simulink model "geometric_control_template"  (R2025b)
settings: Solver=VariableStepAuto  StartTime=0.0  StopTime=30.0  RelTol=1e-3
InitFcn:
  | %% INITIALIZATION
  | 
  | clearvars -except out
  | clc
  | 
  | %% UAV PARAMETERS
  | 
  | mass = 1.2;        % [kg] mass used by controllers
  | mass_real = 1.2;  % [kg] mass used by dynamics
  | 
  | Ib = diag([1.2416 1.2416 2*1.2416]);
  | Ib_ctrl = diag([1.0 0.85 1.80]);
  | %Ib_ctrl = diag([1.2416 1.2416 2*1.2416]);
  | %% SAMPLING TIME
  | 
  | Ts = 0.001;
  | 
  | %% PLANNER
  | 
  | t_iniz = 0;
  | ttot = 22;       % trajectory duration [s]
  | tdead = 8;       % final steady-state time [s]
  | tot_time = ttot + tdead;
  | 
  | % Include exactly t = ttot
  | t1 = 0:Ts:ttot;
  | t_dead = (ttot+Ts):Ts:tot_time;
  | t = [t1, t_dead];
  | 
  | N1 = length(t1);
  | Ndead = length(t_dead);
  | 
  | %% INITIAL CONDITIONS
  | 
  | x0 = 0;
  | y0 = 0;
  | z0 = -1;
  | psi0 = 0;
  | 
  | x0_real = x0;
  | y0_real = y0;
  | z0_real = z0;
  | 
  | pos_0 = [x0_real y0_real z0_real];
  | lin_vel_0 = [0 0 0];
  | w_bb_0 = [0 0 0];
  | 
  | %% SMOOTH NORMALIZED TIME
  | 
  | sigma = t1 / ttot;
  | 
  | % 7th-order smooth step:
  | % s(0)=0, s(1)=1
  | % sdot(0)=sdot(1)=0
  | % sddot(0)=sddot(1)=0
  | % sdddot(0)=sdddot(1)=0
  | 
  | s = 35*sigma.^4 - 84*sigma.^5 + 70*sigma.^6 - 20*sigma.^7;
  | 
  | sdot = (140*sigma.^3 ...
  |       - 420*sigma.^4 ...
  |       + 420*sigma.^5 ...
  |       - 140*sigma.^6) / ttot;
  | 
  | sddot = (420*sigma.^2 ...
  |        - 1680*sigma.^3 ...
  |        + 2100*sigma.^4 ...
  |        - 840*sigma.^5) / ttot^2;
  | 
  | %% DESIRED TRAJECTORY PARAMETERS
  | 
  | Dx = 1.20;
  | Dy = 0.70;
  | Dz = -1.70;
  | 
  | Ay_bump = 0.35;
  | Az_bump = 0.18;
  | 
  | psi_final = deg2rad(25);
  | psi_bump  = deg2rad(6);
  | 
  | %% DESIRED POSITION
  | 
  | x_d = x0 + Dx*s;
  | 
  | y_d = y0 + Dy*s + Ay_bump*sin(2*pi*s);
  | 
  | z_d = z0 + Dz*s + Az_bump*sin(pi*s);
  | 
  | psi_d_traj = psi0 + psi_final*s + psi_bump*sin(pi*s);
  | 
  | %% DERIVATIVES WITH RESPECT TO s
  | 
  | x_s = Dx;
  | x_ss = 0;
  | 
  | y_s = Dy + Ay_bump*2*pi*cos(2*pi*s);
  | y_ss = -Ay_bump*(2*pi)^2*sin(2*pi*s);
  | 
  | z_s = Dz + Az_bump*pi*cos(pi*s);
  | z_ss = -Az_bump*pi^2*sin(pi*s);
  | 
  | psi_s = psi_final + psi_bump*pi*cos(pi*s);
  | psi_ss = -psi_bump*pi^2*sin(pi*s);
  | 
  | %% DESIRED VELOCITY
  | 
  | dot_x_d = x_s .* sdot;
  | dot_y_d = y_s .* sdot;
  | dot_z_d = z_s .* sdot;
  | 
  | dot_psi_d_traj = psi_s .* sdot;
  | 
  | %% DESIRED ACCELERATION
  | 
  | ddot_x_d = x_ss .* sdot.^2 + x_s .* sddot;
  | ddot_y_d = y_ss .* sdot.^2 + y_s .* sddot;
  | ddot_z_d = z_ss .* sdot.^2 + z_s .* sddot;
  | 
  | ddot_psi_d_traj = psi_ss .* sdot.^2 + psi_s .* sddot;
  | 
  | %% ADD FINAL STEADY-STATE PART
  | 
  | x_final = x_d(end);
  | y_final = y_d(end);
  | z_final = z_d(end);
  | psi_final_value = psi_d_traj(end);
  | 
  | p_d = zeros(4, length(t));
  | dot_p_d = zeros(4, length(t));
  | ddot_p_d = zeros(4, length(t));
  | 
  | p_d(1,:) = [x_d, x_final*ones(1, Ndead)];
  | p_d(2,:) = [y_d, y_final*ones(1, Ndead)];
  | p_d(3,:) = [z_d, z_final*ones(1, Ndead)];
  | p_d(4,:) = [psi_d_traj, psi_final_value*ones(1, Ndead)];
  | 
  | dot_p_d(1,:) = [dot_x_d, zeros(1, Ndead)];
  | dot_p_d(2,:) = [dot_y_d, zeros(1, Ndead)];
  | dot_p_d(3,:) = [dot_z_d, zeros(1, Ndead)];
  | dot_p_d(4,:) = [dot_psi_d_traj, zeros(1, Ndead)];
  | 
  | ddot_p_d(1,:) = [ddot_x_d, zeros(1, Ndead)];
  | ddot_p_d(2,:) = [ddot_y_d, zeros(1, Ndead)];
  | ddot_p_d(3,:) = [ddot_z_d, zeros(1, Ndead)];
  | ddot_p_d(4,:) = [ddot_psi_d_traj, zeros(1, Ndead)];
  | 
  | %% DATA FOR SIMULINK
  | 
  | csi_d = p_d(1:3,:);
  | dot_csi_d = dot_p_d(1:3,:);
  | ddot_csi_d = ddot_p_d(1:3,:);
  | 
  | psi_d = p_d(4,:);
  | dot_psi_d = dot_p_d(4,:);
  | ddot_psi_d = ddot_p_d(4,:);
  | 
  | %% DESIRED BODY X-AXIS FROM YAW
  | 
  | xb_des = zeros(3, length(t));
  | 
  | xb_des(1,:) = cos(psi_d);
  | xb_des(2,:) = sin(psi_d);
  | xb_des(3,:) = zeros(1, length(t));
  | 
  | %% EXTERNAL FORCE DISTURBANCE
  | 
  | f_ext = zeros(length(t), 3);
  | 
  | t_f_on = 8;
  | t_f_off = 14;
  | 
  | f_ex_amp = 1.0;    % [N]
  | f_ey_amp = 1.0;    % [N]
  | f_ez_amp = 1.0;    % [N]
  | 
  | t_smooth_f = 0.3;  % [s] smoothing time
  | 
  | w_on_f  = 0.5 * (1 + tanh((t - t_f_on)/t_smooth_f));
  | w_off_f = 0.5 * (1 - tanh((t - t_f_off)/t_smooth_f));
  | 
  | dist_window_f = w_on_f .* w_off_f;
  | 
  | f_ext(:,1) = f_ex_amp * dist_window_f(:);
  | f_ext(:,2) = f_ey_amp * dist_window_f(:);
  | f_ext(:,3) = f_ez_amp * dist_window_f(:);
  | 
  | f_ext_ts = timeseries(f_ext, t(:));
  | 
  | %% EXTERNAL TORQUE DISTURBANCE
  | 
  | tau_ext = zeros(length(t), 3);
  | 
  | t_tau_on = 8;
  | t_tau_off = 14;
  | 
  | tau_ex_amp = 0.0;    % [Nm]
  | tau_ey_amp = 0.5;    % [Nm]
  | tau_ez_amp = 0.0;    % [Nm]
  | 
  | t_smooth_tau = 0.3;  % [s] smoothing time
  | 
  | w_on_tau  = 0.5 * (1 + tanh((t - t_tau_on)/t_smooth_tau));
  | w_off_tau = 0.5 * (1 - tanh((t - t_tau_off)/t_smooth_tau));
  | 
  | dist_window_tau = w_on_tau .* w_off_tau;
  | 
  | tau_ext(:,1) = tau_ex_amp * dist_window_tau(:);
  | tau_ext(:,2) = tau_ey_amp * dist_window_tau(:);
  | tau_ext(:,3) = tau_ez_amp * dist_window_tau(:);
  | 
  | tau_ext_ts = timeseries(tau_ext, t(:));
  | 
  | 
  | %% CHECK
  | 
  | disp("InitFcn completed.")
  | disp("mass = " + string(mass) + " kg")
  | disp("mass_real = " + string(mass_real) + " kg")
  | disp("Simulation time = " + string(tot_time) + " s")
  | disp("Force disturbance: [" + string(f_ex_amp) + ", " + string(f_ey_amp) + ", " + string(f_ez_amp) + "] N")
  | disp("Torque disturbance: [" + string(tau_ex_amp) + ", " + string(tau_ey_amp) + ", " + string(tau_ez_amp) + "] Nm")
undefined symbols (not defined in the file or in its folder): dspblkCoreblockFVToolHelper, gcbh
libraries: robotcorelib x1
settings Model: Creator=fabioruggiero  LastModifiedBy=miche
settings ModelReferenceCC: EnableRefExpFcnMdlSchedulingChecks=on
settings RTWCC: GPUComputeCapability=3.5

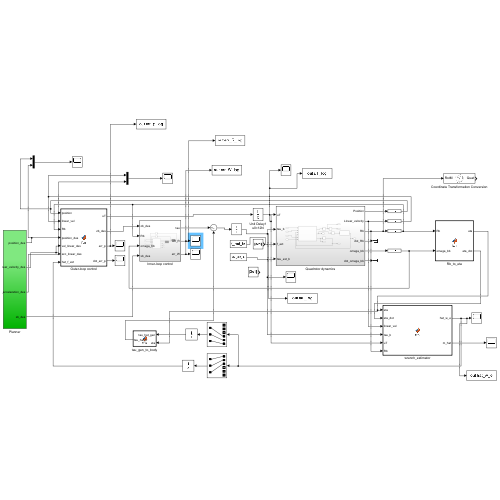
[thumbnail: Simulink's stored preview of the top-level diagram]
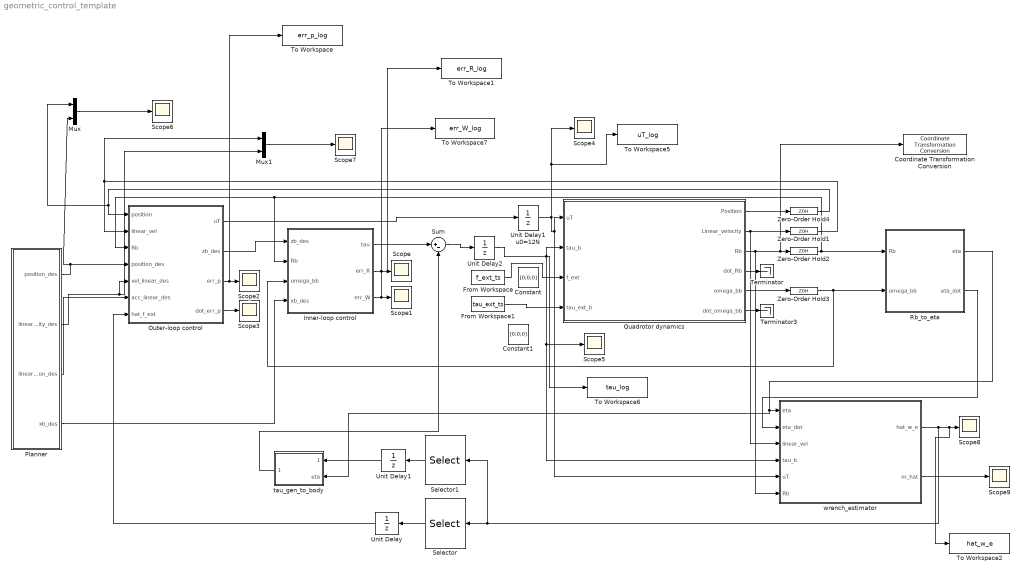
== system geometric_control_template ==
  Constant : Constant  Value=[0;0;0]
  Constant1 : Constant  Value=[0;0;0]
  Coordinate Transformation Conversion : robotcorelib/Coordinate Transformation Conversion  InputRepresentation=Rotation Matrix  InputEulerSequence=ZYX  ShowTrVecInputPort=on  OutputRepresentation=Quaternion  OutputEulerSequence=ZYX  ShowTrVecOutputPort=on  SimulateUsing=Interpreted execution
  From Workspace : FromWorkspace  VariableName=f_ext_ts
  From Workspace1 : FromWorkspace  VariableName=tau_ext_ts
  Inner-loop control : Subsystem
  Mux : Mux  Inputs=2
  Mux1 : Mux  Inputs=2
  Outer-loop control : MATLAB Function  TreatAsAtomicUnit=on
  Planner : Subsystem
  Quadrotor dynamics : Subsystem
  Rb_to_eta : MATLAB Function  TreatAsAtomicUnit=on
  Scope{,1..9} (10 alike) : Scope
      Scope settings: ActiveDisplayYMinimum=-0.020550467345848471  ActiveDisplayYMaximum=0.019993718220872751
      Scope1 settings: ActiveDisplayYMinimum=-0.00025864687025991271  ActiveDisplayYMaximum=0.00043427054129709314
      Scope2 settings: ActiveDisplayYMinimum=-0.0029648084696455505  ActiveDisplayYMaximum=0.02613326914388988  DataLoggingVariableName=ScopeData2
      Scope3 settings: ActiveDisplayYMinimum=-0.00022  ActiveDisplayYMaximum=8E-5  DataLoggingVariableName=ScopeData3
      Scope4 settings: ActiveDisplayYMinimum=11.66747  ActiveDisplayYMaximum=12.03695  DataLoggingVariableName=ScopeData4
      Scope5 settings: ActiveDisplayYMinimum=-5.4477992481437552  ActiveDisplayYMaximum=1.0297199075515178  DataLoggingVariableName=ScopeData5
      Scope6 settings: ActiveDisplayYMinimum=-8.59037  ActiveDisplayYMaximum=7.8245
      Scope7 settings: ActiveDisplayYMinimum=-0.38281946760904528  ActiveDisplayYMaximum=0.16406504710605604  DataLoggingVariableName=ScopeData2
      Scope8 settings: ActiveDisplayYMinimum=-0.0066285466449370889  ActiveDisplayYMaximum=0.0085233543920895938  DataLoggingVariableName=ScopeData6
      Scope9 settings: ActiveDisplayYMinimum=1.1924506191186222  ActiveDisplayYMaximum=1.2266627646008192  DataLoggingVariableName=ScopeData7
  Selector : Selector  InputPortWidth=6  IndexOptions=Index vector (dialog)  Indices=[1 2 3]  OutputSizes=1
  Selector1 : Selector  InputPortWidth=6  IndexOptions=Index vector (dialog)  Indices=[4 5 6]  OutputSizes=1
  Sum : Sum  Inputs=|+-
  Terminator : Terminator
  Terminator3 : Terminator
  To Workspace : ToWorkspace  VariableName=err_p_log  SaveFormat=Timeseries  SampleTime=Ts
  To Workspace1 : ToWorkspace  VariableName=err_R_log  SaveFormat=Timeseries  SampleTime=Ts
  To Workspace2 : ToWorkspace  VariableName=hat_w_e  SaveFormat=Timeseries  SampleTime=Ts
  To Workspace5 : ToWorkspace  VariableName=uT_log  SaveFormat=Timeseries  SampleTime=Ts
  To Workspace6 : ToWorkspace  VariableName=tau_log  SaveFormat=Timeseries  SampleTime=Ts
  To Workspace7 : ToWorkspace  VariableName=err_W_log  SaveFormat=Timeseries  SampleTime=Ts
  Unit Delay : UnitDelay  InitialCondition=[0; 0; 0]  SampleTime=-1  HasFrameUpgradeWarning=on
  Unit Delay1 : UnitDelay  InitialCondition=[0; 0; 0]  SampleTime=-1  HasFrameUpgradeWarning=on
  Unit Delay1 u0=12N : UnitDelay  InitialCondition=12  SampleTime=Ts
  Unit Delay2 : UnitDelay  InitialCondition=[0 0 0]  SampleTime=Ts
  Zero-Order Hold{1..4} (4 alike) : ZeroOrderHold  SampleTime=Ts
  tau_gen_to_body : MATLAB Function  TreatAsAtomicUnit=on
  wrench_estimator : MATLAB Function  TreatAsAtomicUnit=on
  wires:
  Outer-loop control/1(uT) -> Unit Delay1 u0=12N/1
  Unit Delay1 u0=12N/1 -> wrench_estimator/5(uT), Quadrotor dynamics/1(uT), To Workspace5/1, Scope4/1
  Quadrotor dynamics/1(Position) -> Zero-Order Hold4/1
  Quadrotor dynamics/2(Linear_velocity) -> wrench_estimator/3(linear_vel), Zero-Order Hold1/1
  Quadrotor dynamics/3(Rb) -> Coordinate Transformation Conversion/1, Zero-Order Hold2/1, wrench_estimator/6(Rb)
  Quadrotor dynamics/5(omega_bb) -> Zero-Order Hold3/1
  Zero-Order Hold2/1 -> Rb_to_eta/1(Rb), Outer-loop control/3(Rb), Inner-loop control/2(Rb)
  Quadrotor dynamics/4(dot_Rb) -> Terminator/1
  Planner/4(xb_des) -> Inner-loop control/4(xb_des)
  Outer-loop control/3(err_p) -> To Workspace/1, Scope2/1
  Outer-loop control/4(dot_err_p) -> Scope3/1
  Quadrotor dynamics/6(dot_omega_bb) -> Terminator3/1
  Outer-loop control/2(zb_des) -> Inner-loop control/1(zb_des)
  Zero-Order Hold3/1 -> Inner-loop control/3(omega_bb), Rb_to_eta/2(omega_bb)
  Inner-loop control/2(err_R) -> To Workspace1/1, Scope/1
  Inner-loop control/3(err_W) -> To Workspace7/1, Scope1/1
  Planner/1(position_des) -> Mux/2, Outer-loop control/4(position_des)
  Planner/2(linear_velocity_des) -> Mux1/2, Outer-loop control/5(vel_linear_des)
  Planner/3(linear_acceleration_des) -> Outer-loop control/6(acc_linear_des)
  Zero-Order Hold1/1 -> Outer-loop control/2(linear_vel), Mux1/1
  Zero-Order Hold4/1 -> Mux/1, Outer-loop control/1(position)
  Mux/1 -> Scope6/1
  Mux1/1 -> Scope7/1
  Rb_to_eta/1(eta) -> tau_gen_to_body/2(eta), wrench_estimator/1(eta)
  Rb_to_eta/2(eta_dot) -> wrench_estimator/2(eta_dot)
  Unit Delay2/1 -> To Workspace6/1, Quadrotor dynamics/2(tau_b), wrench_estimator/4(tau_b), Scope5/1
  wrench_estimator/2(m_hat) -> Scope9/1
  Selector1/1 -> Unit Delay1/1
  Selector/1 -> Unit Delay/1
  wrench_estimator/1(hat_w_e) -> To Workspace2/1, Scope8/1, Selector1/1, Selector/1
  Unit Delay1/1 -> tau_gen_to_body/1(tau_hat_gen)
  Inner-loop control/1(tau) -> Sum/1
  Sum/1 -> Unit Delay2/1
  From Workspace1/1 -> Quadrotor dynamics/4(tau_ext_b)
  From Workspace/1 -> Quadrotor dynamics/3(f_ext)
  Unit Delay/1 -> Outer-loop control/7(hat_f_ext)
  tau_gen_to_body/1(tau_hat_b) -> Sum/2

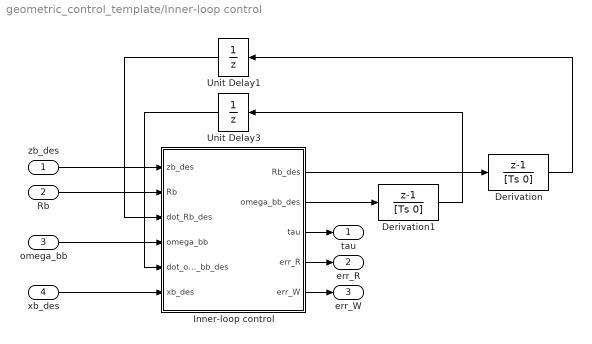
== system geometric_control_template/Inner-loop control ==
  zb_des : Inport
  Rb : Inport  Port=2
  omega_bb : Inport  Port=3
  xb_des : Inport  Port=4
  Derivation : DiscreteTransferFcn  LoadFcn=dspblkCoreblockFVToolHelper(gcbh,'load');  Numerator=[1 -1]  Denominator=[Ts 0]  InitialStates=[1 0 0;0 1 0;0 0 1]  SampleTime=Ts
      settings: CopyFcn=dspblkCoreblockFVToolHelper(gcbh,'copy');  DeleteFcn=dspblkCoreblockFVToolHelper(gcbh,'close');  ModelCloseFcn=dspblkCoreblockFVToolHelper(gcbh,'close');  PreSaveFcn=dspblkCoreblockFVToolHelper(gcbh,'presave');  PostSaveFcn=dspblkCoreblockFVToolHelper(gcbh,'postsave');  CloseFcn=dspblkCoreblockFVToolHelper(gcbh,'close');
  Derivation1 : DiscreteTransferFcn  Numerator=[1 -1]  Denominator=[Ts 0]  InitialStates=[0 0 0]  SampleTime=Ts
  Inner-loop control : MATLAB Function  TreatAsAtomicUnit=on
  Unit Delay1 : UnitDelay  InitialCondition=eye(3)  SampleTime=Ts
  Unit Delay3 : UnitDelay  InitialCondition=[0 0 0]  SampleTime=Ts
  tau : Outport
  err_R : Outport  Port=2
  err_W : Outport  Port=3
  wires:
  xb_des/1 -> Inner-loop control/6(xb_des)
  Inner-loop control/4(err_R) -> err_R/1
  Rb/1 -> Inner-loop control/2(Rb)
  Inner-loop control/3(tau) -> tau/1
  Unit Delay1/1 -> Inner-loop control/3(dot_Rb_des)
  Derivation1/1 -> Unit Delay3/1
  Inner-loop control/5(err_W) -> err_W/1
  Unit Delay3/1 -> Inner-loop control/5(dot_omega_bb_des)
  Derivation/1 -> Unit Delay1/1
  zb_des/1 -> Inner-loop control/1(zb_des)
  omega_bb/1 -> Inner-loop control/4(omega_bb)
  Inner-loop control/1(Rb_des) -> Derivation/1
  Inner-loop control/2(omega_bb_des) -> Derivation1/1

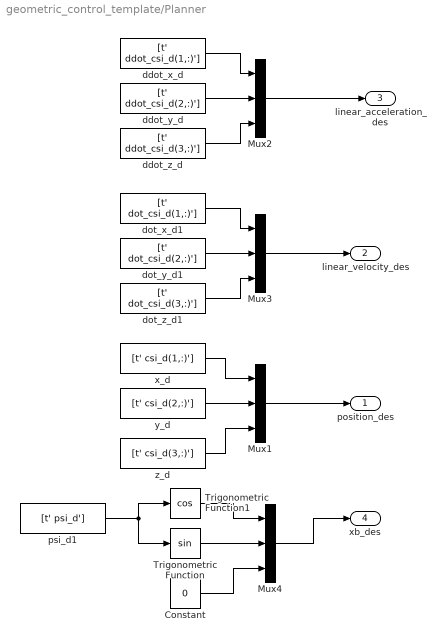
== system geometric_control_template/Planner ==
  Constant : Constant  Value=0
  Mux{1..4} (4 alike) : Mux  Inputs=3
  Trigonometric Function : Trigonometry
  Trigonometric Function1 : Trigonometry  Operator=cos
  ddot_x_d : FromWorkspace  VariableName=[t' ddot_csi_d(1,:)']  SampleTime=Ts
  ddot_y_d : FromWorkspace  VariableName=[t' ddot_csi_d(2,:)']  SampleTime=Ts
  ddot_z_d : FromWorkspace  VariableName=[t' ddot_csi_d(3,:)']  SampleTime=Ts
  dot_x_d1 : FromWorkspace  VariableName=[t' dot_csi_d(1,:)']  SampleTime=Ts
  dot_y_d1 : FromWorkspace  VariableName=[t' dot_csi_d(2,:)']  SampleTime=Ts
  dot_z_d1 : FromWorkspace  VariableName=[t' dot_csi_d(3,:)']  SampleTime=Ts
  psi_d1 : FromWorkspace  VariableName=[t' psi_d']  SampleTime=Ts
  x_d : FromWorkspace  VariableName=[t' csi_d(1,:)']  SampleTime=Ts
  y_d : FromWorkspace  VariableName=[t' csi_d(2,:)']  SampleTime=Ts
  z_d : FromWorkspace  VariableName=[t' csi_d(3,:)']  SampleTime=Ts
  position_des : Outport
  linear_velocity_des : Outport  Port=2
  linear_acceleration_des : Outport  Port=3
  xb_des : Outport  Port=4
  wires:
  y_d/1 -> Mux1/2
  z_d/1 -> Mux1/3
  x_d/1 -> Mux1/1
  ddot_y_d/1 -> Mux2/2
  ddot_z_d/1 -> Mux2/3
  ddot_x_d/1 -> Mux2/1
  Mux2/1 -> linear_acceleration_des/1
  Mux1/1 -> position_des/1
  dot_y_d1/1 -> Mux3/2
  dot_z_d1/1 -> Mux3/3
  dot_x_d1/1 -> Mux3/1
  Mux3/1 -> linear_velocity_des/1
  Mux4/1 -> xb_des/1
  Trigonometric Function/1 -> Mux4/2
  psi_d1/1 -> Trigonometric Function/1, Trigonometric Function1/1
  Trigonometric Function1/1 -> Mux4/1
  Constant/1 -> Mux4/3

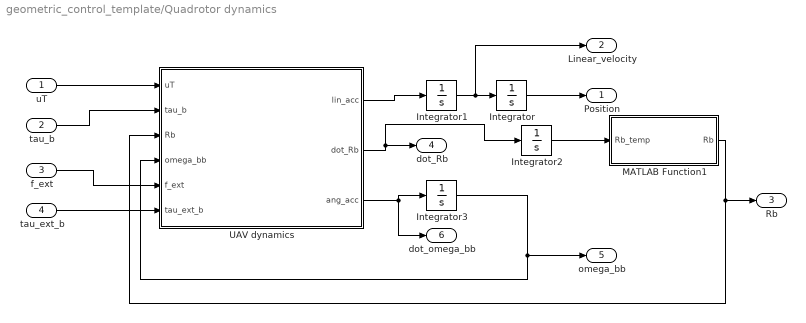
== system geometric_control_template/Quadrotor dynamics ==
  uT : Inport
  tau_b : Inport  Port=2
  f_ext : Inport  Port=3
  tau_ext_b : Inport  Port=4
  Integrator : Integrator  InitialCondition=pos_0
  Integrator1 : Integrator  InitialCondition=lin_vel_0
  Integrator2 : Integrator  InitialCondition=[1 0 0; 0 1 0;0 0 1]
  Integrator3 : Integrator  InitialCondition=w_bb_0
  MATLAB Function1 : MATLAB Function  TreatAsAtomicUnit=on
  UAV dynamics : MATLAB Function  TreatAsAtomicUnit=on
  Position : Outport
  Linear_velocity : Outport  Port=2
  Rb : Outport  Port=3
  dot_Rb : Outport  Port=4
  omega_bb : Outport  Port=5
  dot_omega_bb : Outport  Port=6
  wires:
  tau_b/1 -> UAV dynamics/2(tau_b)
  Integrator/1 -> Position/1
  UAV dynamics/3(ang_acc) -> Integrator3/1, dot_omega_bb/1
  UAV dynamics/1(lin_acc) -> Integrator1/1
  uT/1 -> UAV dynamics/1(uT)
  Integrator1/1 -> Linear_velocity/1, Integrator/1
  Integrator3/1 -> UAV dynamics/4(omega_bb), omega_bb/1
  UAV dynamics/2(dot_Rb) -> Integrator2/1, dot_Rb/1
  MATLAB Function1/1(Rb) -> Rb/1, UAV dynamics/3(Rb)
  Integrator2/1 -> MATLAB Function1/1(Rb_temp)
  f_ext/1 -> UAV dynamics/5(f_ext)
  tau_ext_b/1 -> UAV dynamics/6(tau_ext_b)

== matlab function geometric_control_template/Rb_to_eta ==
  data: Rb input; eta output; omega_bb input; eta_dot output
function [eta, eta_dot] = fcn(Rb, omega_bb)

r31 = Rb(3,1);
r31 = max(min(r31,1),-1);

phi   = atan2(Rb(3,2), Rb(3,3));
theta = -asin(r31);
psi   = atan2(Rb(2,1), Rb(1,1));

eta = [phi; theta; psi];

cphi = cos(phi);
sphi = sin(phi);
cth  = cos(theta);
sth  = sin(theta);

Q = [1, 0, -sth;
     0, cphi, cth*sphi;
     0, -sphi, cth*cphi];

eta_dot = Q \ omega_bb;

== matlab function geometric_control_template/Quadrotor dynamics/UAV dynamics ==
  data: uT input size=1; tau_b input size=3; lin_acc output size=3; Rb input size=[3,3]; omega_bb input size=3; dot_Rb output size=[3,3]; ang_acc output size=3; mass parameter size=1; Ib parameter size=[3,3]; f_ext input; tau_ext_b input
function [lin_acc, dot_Rb, ang_acc] = fcn(uT,tau_b,Rb,omega_bb,mass, Ib, f_ext, tau_ext_b)

e3 = [0; 0; 1];

uT = double(uT);
tau_b = reshape(tau_b, [3 1]);
Rb = reshape(Rb, [3 3]);
omega_bb = reshape(omega_bb, [3 1]);
f_ext = reshape(f_ext, [3 1]);
tau_ext_b = reshape(tau_ext_b, [3 1]);

lin_acc = 9.81*e3 - (uT/mass)*Rb*e3 + f_ext/mass;

dot_Rb = Rb*skew(omega_bb);

ang_acc = Ib \ (-skew(omega_bb)*Ib*omega_bb + tau_b + tau_ext_b);

end


function S = skew(v)

v = reshape(v, [3 1]);

S = [   0   -v(3)  v(2);
      v(3)    0   -v(1);
     -v(2)  v(1)    0];

end

== matlab function geometric_control_template/Outer-loop control ==
  data: position input size=3; uT output size=1; linear_vel input size=3; Rb input size=[3,3]; zb_des output size=3; mass_real parameter size=1; position_des input size=3; vel_linear_des input size=3; acc_linear_des input size=3; err_p output size=3; dot_err_p output size=3; hat_f_ext input
function [uT, zb_des, err_p, dot_err_p] = fcn(position, linear_vel, Rb, mass_real, ...
    position_des, vel_linear_des, acc_linear_des, hat_f_ext)

% position: linear position measure
% linear_vel: linear velocity measure
% Rb: current rotation matrix
% mass: mass of the UAV
% position_des: desired linear position from the planner
% vel_linear_des: desired linear velocity from the planner
% acc_linear_des: desired linear acceleration from the planner
% hat_w_e: estimated external wrench
%          hat_w_e(1:3) = estimated external force in world frame
%          hat_w_e(4:6) = estimated angular disturbance, not used here
%
% uT: commanded total thrust
% zb_des: desired z-axis of the body frame
% err_p: position error
% dot_err_p: derivative of position error

% === Constants ===
g = 9.81;
e3 = [0; 0; 1];



% === Controller gains ===
Kp = diag([40, 40, 40]);
Kv = diag([20, 20, 20]);

% === Errors ===
err_p = position - position_des;
dot_err_p = linear_vel - vel_linear_des;

% === External force estimate ===
f_hat = hat_f_ext(1:3);

% === Nominal desired force vector ===
A = -Kp * err_p ...
    -Kv * dot_err_p ...
    -mass_real * g * e3 ...
    +mass_real * acc_linear_des;

% === Compensation of estimated external force ===
A_comp = A - f_hat;

% === Safety against division by zero ===
A_norm = norm(A_comp);

if A_norm < 1e-6
    A_comp = -mass_real * g * e3;
    A_norm = norm(A_comp);
end

% === Total thrust ===
uT = -A_comp' * (Rb * e3);

% === Desired body z-axis ===
zb_des = -A_comp / A_norm;

end

== matlab function geometric_control_template/Inner-loop control/Inner-loop control ==
  data: Rb_des output size=[3,3]; omega_bb_des output size=3; tau output size=3; zb_des input size=3; Rb input size=[3,3]; dot_Rb_des input size=[3,3]; omega_bb input size=3; dot_omega_bb_des input size=3; xb_des input size=3; Ib_ctrl parameter size=[3,3]; err_R output size=3; err_W output size=3
function [Rb_des,omega_bb_des,tau,err_R,err_W] = fcn(zb_des,Rb,dot_Rb_des,omega_bb,dot_omega_bb_des,xb_des,Ib_ctrl)

%% WRITE HERE THE INNER-LOOP CONTROL
% zb_des: desired z-axis of the body frame
% Rb: current rotation matrix
% dot_Rb_des: time-derivative of the desired rotation matrix
% omega_bb: current angular velocity expressed in the body frame
% dot_omega_bb_des: desired angular acceleration expressed in the body
% frame
% xb_des: desired x-axis of the body frame form the planner
% Ib: inertia matrix of the UAV with respect to the body frame
% ---
% Rb_des: desired rotation matrix
% omega_bb_des: desired angular velocity expressed in the body frame (given
% below as a hint)
% tau: commanded control torque
% err_R: rotational error in SO(3)
% err_W: angular velocity error in SO(3)

% === RICOSTRUZIONE DI Rb_des ===
yb_des = skew(zb_des) * xb_des;
yb_des = yb_des / norm(yb_des);

xb_des_ortho = skew(yb_des) * zb_des;
Rb_des = [xb_des_ortho, yb_des, zb_des];

omega_bb_des = wedge(Rb_des'*dot_Rb_des);

% === Errore di orientamento (SO(3)) ===
error_matrix = (Rb_des' * Rb - Rb' * Rb_des);
err_R = 0.5 * wedge(error_matrix);    % vee operatore

% === Errore di velocità angolare ===
err_W = omega_bb - Rb' * Rb_des * omega_bb_des;

% === Guadagni del controllore ===
KR = diag([10, 10, 8]);
Komega = diag([6, 6, 5]);


% === Calcolo del momento di controllo tau ===
tau = -KR * err_R - Komega * err_W + skew(omega_bb) * Ib_ctrl * omega_bb - Ib_ctrl * (skew(omega_bb) * Rb' * Rb_des * omega_bb_des - Rb' * Rb_des * dot_omega_bb_des);





end

function S = skew(v)
if(numel(v)~= 1)
S= [0 -v(3) v(2); 
    v(3) 0 -v(1);
    -v(2) v(1) 0];
else
S= zeros(3);
end
end

function v = wedge(S)
v1 = S(3,2);
v2 = S(1,3);
v3 = S(2,1);
v = [v1 v2 v3]';
end

== matlab function geometric_control_template/Quadrotor dynamics/MATLAB Function1 ==
  data: Rb_temp input; Rb output
function Rb = fcn(Rb_temp)
    [U,S,V] = svd(Rb_temp);
    sigma = det(U*V');
    S_ = diag([1 1 sigma]);

    Rb = U*S_*V';
end

== matlab function geometric_control_template/tau_gen_to_body ==
  data: tau_hat_gen input; tau_hat_b output; eta input
function tau_hat_b = fcn(tau_hat_gen, eta)

tau_hat_gen = reshape(tau_hat_gen, [3 1]);
eta = reshape(eta, [3 1]);

phi = eta(1);
theta = eta(2);

cphi = cos(phi);
sphi = sin(phi);
cth  = cos(theta);
sth  = sin(theta);

Q = [1, 0, -sth;
     0, cphi, cth*sphi;
     0, -sphi, cth*cphi];

tau_hat_b_col = Q' \ tau_hat_gen;



% Output as 3-element row/vector, not [3x1] matrix
tau_hat_b = tau_hat_b_col.';

end

== matlab function geometric_control_template/wrench_estimator ==
  settings: updateMethod=DISCRETE
  data: eta input; hat_w_e output; eta_dot input; linear_vel input; tau_b input; uT input; Rb input; m_hat output
function [hat_w_e, m_hat] = fcn(eta, eta_dot, linear_vel, tau_b, uT, Rb)

% External wrench estimator
% hat_w_e = [f_ext_world; tau_ext_generalized]

Ts = 0.001;

m = 1.2;
J = diag([1.2416 1.2416 2*1.2416]);
g = 9.81;
e3 = [0; 0; 1];

% ==========================
% Estimator parameters
% ==========================
r = 3;           % try: 1, 2, 3, 5, 10
omega_c = 12;    % cutoff frequency [rad/s]

RMAX = 20;
r = max(1, min(round(r), RMAX));

% ==========================
% Compute gains K from (s + omega_c)^r
% ==========================
K = zeros(1, RMAX);
c = zeros(1, RMAX);

for j = 0:RMAX-1
    if j <= r-1
        c(j+1) = binom_coeff(r,j) * omega_c^(r-j);
    end
end

K(r) = c(r);

for j = RMAX-1:-1:1
    if j < r
        prod_next = 1;
        for k = j+1:r
            prod_next = prod_next * K(k);
        end
        K(j) = c(j) / prod_next;
    end
end

% ==========================
% Force dimensions
% ==========================
eta        = reshape(eta,        [3 1]);
eta_dot    = reshape(eta_dot,    [3 1]);
linear_vel = reshape(linear_vel, [3 1]);
tau_b      = reshape(tau_b,      [3 1]);
Rb         = reshape(Rb,         [3 3]);

hat_w_e = zeros(6,1);
m_hat = 0;

persistent gamma hat_w_prev int_hat_w int_model eta_prev initialized

if isempty(initialized)
    gamma = zeros(6, RMAX);
    hat_w_prev = zeros(6,1);
    int_hat_w = zeros(6,1);
    int_model = zeros(6,1);
    eta_prev = eta;
    initialized = true;
end

% ==========================
% Model matrices
% ==========================
Q = Q_matrix(eta);
C = C_matrix(eta, eta_dot, eta_prev, Ts, J);
M_eta = Q' * J * Q;

% Generalized momentum
q = [m*eye(3), zeros(3,3);
     zeros(3,3), M_eta] * [linear_vel; eta_dot];

% Nominal model term
upper = m*g*e3 - uT * Rb * e3;
lower = C' * eta_dot + Q' * tau_b;

model_term = [upper; lower];

% ==========================
% Integrals
% ==========================
int_hat_w = int_hat_w + hat_w_prev * Ts;
int_model = int_model + model_term * Ts;

% ==========================
% r-th order estimator
% ==========================
gamma(:,1) = K(1) * (q - int_hat_w - int_model);

for i = 2:RMAX
    if i <= r
        gamma(:,i) = gamma(:,i) + ...
            K(i) * (gamma(:,i-1) - hat_w_prev) * Ts;
    end
end

hat_w_e = gamma(:,r);
hat_w_prev = hat_w_e;

% Mass estimate
m_hat = (uT * Rb(3,:) * e3 - hat_w_e(3)) / g;

eta_prev = eta;

end


function Q = Q_matrix(eta)

phi = eta(1);
theta = eta(2);

cphi = cos(phi);
sphi = sin(phi);
cth  = cos(theta);
sth  = sin(theta);

Q = [1, 0, -sth;
     0, cphi, cth*sphi;
     0, -sphi, cth*cphi];

end


function C = C_matrix(eta, eta_dot, eta_prev, Ts, J)

Q = Q_matrix(eta);
Q_prev = Q_matrix(eta_prev);

Q_dot = (Q - Q_prev) / Ts;
omega = Q * eta_dot;

C = Q' * skew(omega) * J * Q + Q' * J * Q_dot;

end


function S = skew(v)

v = reshape(v, [3 1]);

S = [   0   -v(3)  v(2);
      v(3)    0   -v(1);
     -v(2)  v(1)    0];

end


function b = binom_coeff(n,k)

b = 1;

if k < 0 || k > n
    b = 0;
else
    for i = 1:k
        b = b * (n - k + i) / i;
    end
end

end
